simulink model "controller"  (R2021b)
settings: Solver=VariableStepAuto  StartTime=0.0  StopTime=5  RelTol=1e-3
values from neighbouring files (symbols this model uses):
  K_b = 1/4.6027    (= 0.217263779955)    [controller_m.m]
  Kd = 0.4    [controller_m.m]
  Ki = 0.05    [controller_m.m]
  Kp = 2.4    [controller_m.m]
  tau_m = 0.22    [controller_m.m]
settings Model: Creator=Dalton  LastModifiedBy=Dalton

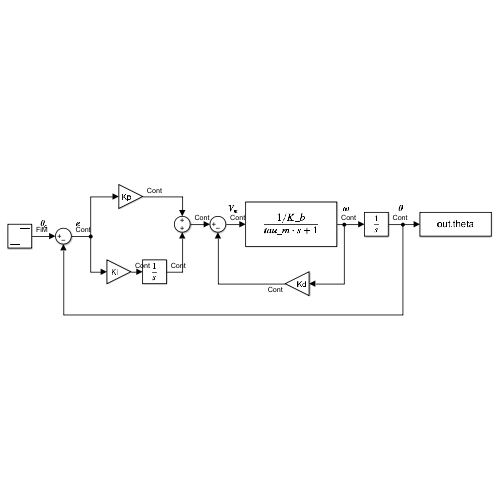
[thumbnail: Simulink's stored preview of the top-level diagram]
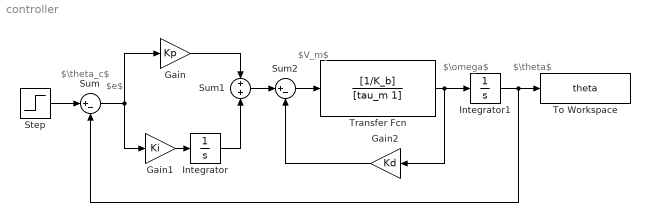
== system controller ==
  note: $V_m$
  note: $\omega$
  note: $\theta$
  note: $\theta_c$
  note: $e$
  Gain : Gain  Gain=Kp
  Gain1 : Gain  Gain=Ki
  Gain2 : Gain  Gain=Kd
  Integrator : Integrator
  Integrator1 : Integrator
  Step : Step  SampleTime=0
  Sum : Sum  Inputs=|+-
  Sum1 : Sum
  Sum2 : Sum  Inputs=|+-
  To Workspace : ToWorkspace  VariableName=theta  SampleTime=-1
  Transfer Fcn : TransferFcn  Numerator=[1/K_b]  Denominator=[tau_m 1]
  wires:
  Transfer Fcn/1 -> Integrator1/1, Gain2/1
  Step/1 -> Sum/1
  Sum/1 -> Gain1/1, Gain/1
  Gain1/1 -> Integrator/1
  Gain/1 -> Sum1/1
  Integrator/1 -> Sum1/2
  Integrator1/1 -> To Workspace/1, Sum/2
  Sum1/1 -> Sum2/1
  Sum2/1 -> Transfer Fcn/1
  Gain2/1 -> Sum2/2
